simulink model "Motor_Model"  (R2025b)
settings: Solver=VariableStepAuto  StartTime=0.0  StopTime=10.0  RelTol=1e-3
settings Model: Creator=joshc  LastModifiedBy=joshc

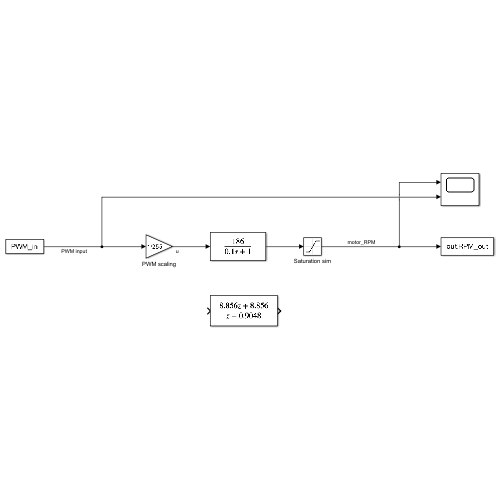
[thumbnail: Simulink's stored preview of the top-level diagram]
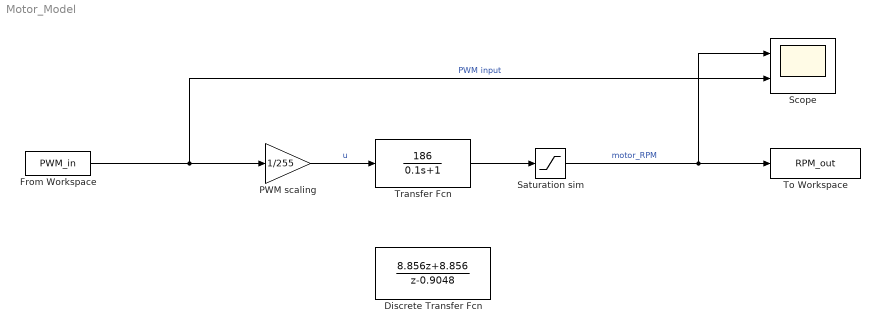
== system Motor_Model ==
  Discrete Transfer Fcn : DiscreteTransferFcn  Numerator=[8.856,8.856]  Denominator=[1, -0.9048]
  From Workspace : FromWorkspace  VariableName=PWM_in  SampleTime=-1  Interpolate=off  ZeroCross=off  OutputAfterFinalValue=Holding final value
  PWM scaling : Gain  Gain=1/255
  Saturation sim : Saturate  UpperLimit=186  LowerLimit=0
  Scope : Scope  NumInputPorts=2
      settings: ActiveDisplayYMinimum=21.483969044386214  ActiveDisplayYMaximum=264.658595655016
  To Workspace : ToWorkspace  VariableName=RPM_out  SampleTime=0.01
      settings: Save2DSignal=2-D array (concatenate along first dimension)
  Transfer Fcn : TransferFcn  Numerator=[186]  Denominator=[0.1 1]
  wires:
  PWM scaling/1 -> Transfer Fcn/1  "u"
  Transfer Fcn/1 -> Saturation sim/1
  Saturation sim/1 -> Scope/1, To Workspace/1  "motor_RPM"
  From Workspace/1 -> Scope/2, PWM scaling/1  "PWM input"
